simulink model "TraditionalStarterGenerator"  (R2024b)
settings: Solver=VariableStepAuto  StartTime=0.0  StopTime=20  MaxStep=1  RelTol=1e-3  EnableMultiTasking=on
undefined symbols (not defined in the file or in its folder): DiscIntNeverNeededParam
libraries: fl_lib x47, fl_ps_legacy_lib x26, ee_lib x25, nesl_utility x17, sdl_lib x1, SignalEditorBlockLib x1
(part 1 of 2)
CloseFcn:
  | try,close(h1_AutomotiveElectrical),end
  | clear h1_AutomotiveElectrical
  | 
  | clear simlog_AutomotiveElectrical
  | clear logsout_AutomotiveElectrical
  | clear tout
Description:
  | Automotive Electrical System
settings Model: Creator=The MathWorks, Inc.  LastModifiedBy=Ujjal.Ghosh
settings SolverCC: AlgebraicLoopSolver=TrustRegion  MaxZcPerStep=1
settings DataIOCC: LimitDataPoints=on  MaxDataPoints=15000  SaveFormat=Array  ReturnWorkspaceOutputs=off  SignalLoggingName=logsout_AutomotiveElectrical
settings OptimizationCC: ReuseModelBlockBuffer=off  ExpressionDepthLimit=2147483647  LifeSpan=inf
settings DebuggingCC: UnderspecifiedInitializationDetection=Classic  MergeDetectMultiDrivingBlocksExec=none  SolverPrmCheckMsg=warning  FcnCallInpInsideContextMsg=warning  UnconnectedInputMsg=warning  UnconnectedOutputMsg=warning  UnconnectedLineMsg=warning  AllowSymbolicDim=off  StateNameClashWarn=warning  SFUnexpectedBacktrackingDiag=warning  SFNoUnconditionalDefaultTransitionDiag=warning  SFExecutionAtInitializationDiag=none  ArithmeticOperatorsInVariantConditions=warning
settings HardwareCC: ProdBitPerPointer=32  ProdBitPerSizeT=32  ProdBitPerPtrDiffT=32  ProdLargestAtomicFloat=None  ProdIntDivRoundTo=Undefined  ProdEndianess=Unspecified  ProdWordSize=32  ProdHWDeviceType=32-bit Generic
settings ModelReferenceCC: EnableRefExpFcnMdlSchedulingChecks=on  PropagateSignalLabelsOutOfModel=off
settings SFSimCC: SimUseLocalCustomCode=off  CustomCodeUndefinedFunction=UseInterfaceOnly
settings RTWCC: RTWUseLocalCustomCode=off  GPUComputeCapability=3.5  DLArmComputeVersion=19.05
settings CodeAppCC: StateflowObjectComments=on
settings GRTTargetCC: TargetLangStandard=C89/C90 (ANSI)  CombineOutputUpdateFcns=off  GRTInterface=on
settings ConfigComp: CovMetricSettings=dw  CovSaveCumulativeToWorkspaceVar=on  CovSaveSingleToWorkspaceVar=on  CovExternalEMLEnable=off  CovSFcnEnable=off
settings SimscapeCC: SimscapeLogType=all  SimscapeLogSimulationStatistics=on  SimscapeLogName=simlog_AutomotiveElectrical  SimscapeLogDataHistory=15000

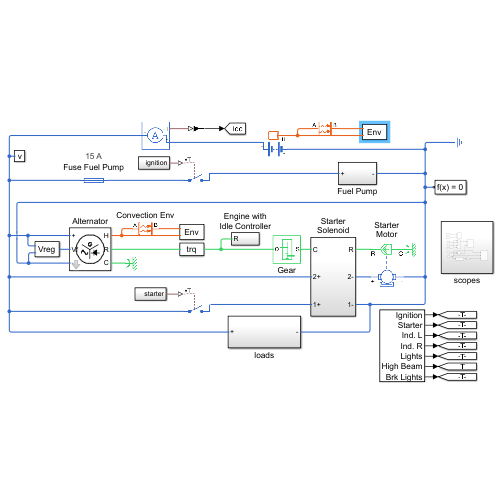
[thumbnail: Simulink's stored preview of the top-level diagram]
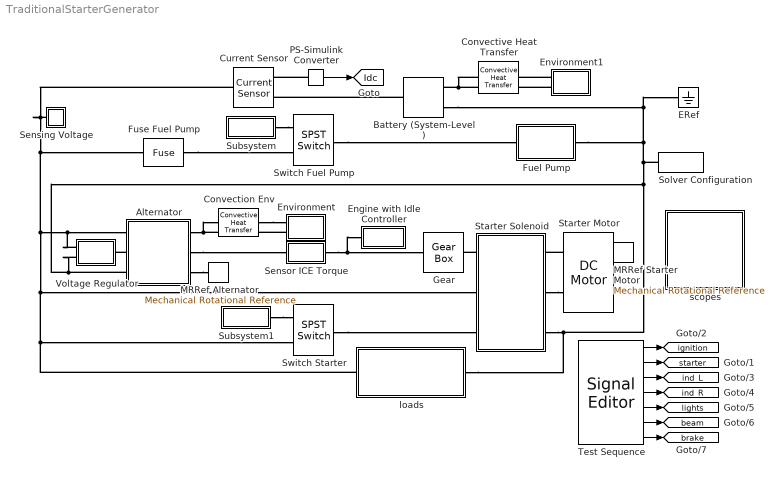
== system TraditionalStarterGenerator ==
  Alternator : Subsystem  mask(Abstracted Alternator){Kv=0.00125, Vmin=0.7, R=0.085, J=3*385, T0=25}
      mask prompts: Kv "Back emf constant (V/rpm)"; Vmin "Rectifier diode total forward voltage drop (V)"; R "Stator resistance represented on DC side (Ohm)"; J "Thermal mass (J/K)"; T0 "Initial temperature (deg C)"
      mask Display:
      | plot([287.470623152331;286.906458966957;285.219399620346;282.425692416244;278.552242282225;273.63635266052;267.725366255486;260.876209097478;253.154842314056;244.635626888274;235.40060752176;225.538722499386;215.144947164975;204.319379256811;193.166274911708;181.793044621416;170.309218810871;158.825393000326;147.452162710034;136.299058364931;125.473490456767;115.079715122356;105.217830099983;95.9828107334681;87.4635953076864;79.7422285242648;72.8930713662563;66.9820849612226;62.066195339518;58.1927452054981;55.3990380013969;53.7119786547854;53.147814469412;53.7119786547854;55.3990380013969;58.1927452054983;62.0661953395182;66.9820849612228;72.8930713662566;79.7422285242652;87.4635953076867;95.9828107334684;105.217830099983;115.079715122356;125.473490456768;136.299058364931;147.452162710034;158.825393000326;170.309218810871;181.793044621417;193.166274911708;204.319379256811;215.144947164975;225.538722499386;235.40060752176;244.635626888274;253.154842314056;260.876209097477;267.725366255486;273.63635266052;278.552242282224;282.425692416244;285.219399620346;286.906458966957;287.470623152331;287.470623152331;287.470623152331], [170.309218810871;158.825393000326;147.452162710034;136.299058364931;125.473490456768;115.079715122356;105.217830099983;95.9828107334682;87.4635953076864;79.7422285242649;72.8930713662564;66.9820849612227;62.0661953395181;58.1927452054982;55.3990380013969;53.7119786547854;53.147814469412;53.7119786547854;55.3990380013969;58.1927452054982;62.0661953395181;66.9820849612227;72.8930713662565;79.742228524265;87.4635953076865;95.9828107334683;105.217830099983;115.079715122356;125.473490456768;136.299058364931;147.452162710034;158.825393000326;170.309218810872;181.793044621417;193.166274911709;204.319379256812;215.144947164975;225.538722499387;235.40060752176;244.635626888275;253.154842314056;260.876209097478;267.725366255486;273.63635266052;278.552242282225;282.425692416244;285.219399620346;286.906458966957;287.470623152331;286.906458966957;285.219399620346;282.425692416244;278.552242282225;273.63635266052;267.725366255486;260.876209097478;253.154842314056;244.635626888275;235.40060752176;225.538722499387;215.144947164975;204.319379256812;193.166274911709;181.793044621417;170.309218810872;170.309218810871;170.309218810871])
      | patch([5.6843418860808e-14;340.618437621743;340.618437621743;0;5.6843418860808e-14;0.472425017505941;0.472425017505941;340.146012604237;340.146012604237;0.472425017505941;5.6843418860808e-14], [340.618437621743;340.618437621743;0;5.6843418860808e-14;340.618437621743;340.146012604237;0.472425017505941;0.472425017505941;340.146012604237;340.146012604237;340.618437621743], [1;1;1])
      | plot([170.309218810871;170.309218810871], [170.309218810871;96.6109160799534])
      | plot([234.118091175333;170.309218810871], [207.15837017633;170.309218810871])
      | plot([169.868288794532;106.059416430071], [169.553338782862;206.465480150655])
      | plot([249.67662175186;181.647419231013], [141.963717760518;141.963717760518])
      | patch([227.000220911577;227.000220911577;204.323820071295;227.000220911577], [122.121867025271;161.805568495765;141.963717760518;122.121867025271], [0;0;0])
      | plot([227.000220911577;227.000220911577;204.323820071295;227.000220911577], [122.121867025271;161.805568495765;141.963717760518;122.121867025271])
      | plot([173.143768915907;184.481969336048], [204.323820071295;204.323820071295])
      | plot([204.323820071295;204.323820071295], [161.805568495765;122.121867025271])
      | plot([178.812869125977;178.749879123643;178.560909116641;178.308949107304;177.993999095634;177.490079076961;176.923169055954;176.356259034947;175.600379006937;174.844498978928;173.96263894625;172.89180890657;171.694998862222;170.309218810871;168.923438759521;167.600648710504;166.529818670824;165.710948640481;165.08104861714;164.577128598467;164.136198582128;163.758258568123;163.317328551784;162.687428528443;161.994538502768;161.049688467756;160.04184843041;158.97101839073;157.90018835105;157.207298325375;156.703378306702;156.451418297365;156.388428295031;156.388428295031;156.388428295031;156.388428295031;156.388428295031;156.325438292697;156.199458288029;156.136468285695;156.199458288029;156.325438292697;156.388428295031;156.388428295031;156.388428295031;156.388428295031;156.388428295031;156.451418297365;156.703378306702;157.207298325375;157.90018835105;158.97101839073;160.04184843041;161.049688467756;161.994538502768;162.687428528443;163.317328551784;163.758258568123;164.199188584462;164.577128598467;165.08104861714;165.710948640481;166.529818670824;167.600648710504;168.923438759521;170.309218810871;171.883968869224;173.143768915907;174.088618950918;174.781508976594;175.159448990598;175.537389004603;175.78934901394;176.167289027944;176.608219044283;177.238119067624;178.056989097968;178.812869125977;179.190809139982;179.442769149318;179.631739156321;179.757719160989;179.883699165657;179.883699165657;179.883699165657;179.883699165657;179.820709163323;179.694729158655;179.631739156321;179.505759151653;179.379779146984;179.253799142316;179.127819137648;179.064829135314;178.938849130645;178.875859128311;178.812869125977], [218.496570596471;218.62255060114;218.811520608142;219.189460622147;219.69338064082;220.323280664161;220.953180687502;221.646070713177;222.275970736519;222.842880757526;223.346800776199;223.787730792537;224.039690801874;224.165670806542;224.039690801874;223.850720794872;223.535770783201;223.283810773864;223.031850764528;222.779890755192;222.527930745855;222.212980734184;221.898030722514;221.520090708509;220.953180687502;220.323280664161;219.441420631483;218.496570596471;217.299760552123;216.291920514777;215.536040486768;215.032120468095;214.717170456424;214.465210447088;214.213250437751;213.898300426081;213.331390405074;212.51252037473;211.378700332716;209.992920281366;208.607140230015;207.473320188001;206.654450157657;206.08754013665;205.77259012498;205.520630115643;205.268670106307;204.953720094636;204.449800075963;203.693920047954;202.686080010608;201.48926996626;200.544419931248;199.66255989857;199.032659875229;198.465749854222;198.087809840217;197.772859828547;197.457909816876;197.20594980754;196.953989798203;196.702029788867;196.45006977953;196.13511976786;195.946149760857;195.820169756189;195.946149760857;196.261099772528;196.702029788867;197.079969802871;197.52089981921;197.961829835549;198.402759851888;198.906679870561;199.410599889234;200.040499912575;200.73338993825;201.48926996626;201.867209980264;202.182159991935;202.497110003606;202.749070012942;203.001030022278;203.190000029281;203.378970036283;203.504950040951;203.63093004562;203.756910050288;203.882890054956;203.94588005729;204.071860061958;204.134850064293;204.197840066627;204.260830068961;204.260830068961;204.323820071295;204.323820071295])
      | plot([98.8785561639816;98.9415461663157;99.0045361686498;99.1935061756522;99.5084561873228;99.8863962013275;100.327326217666;100.831246236339;101.46114625968;102.091046283022;102.783936308697;103.60280633904;104.421676369384;105.366526404396;106.374366441742;107.57117648609;108.830976532772;110.216756584123;111.602536635473;112.92532668449;114.059146726504;115.003996761516;115.696886787191;116.200806805864;116.578746819869;116.830706829205;117.082666838542;117.271636845544;117.586586857215;117.964526871219;118.531436892226;119.224326917902;120.232166955248;121.428976999596;122.814757050946;124.389507109299;125.964257167652;127.350037219003;128.546847263351;129.554687300697;130.247577326372;130.814487347379;131.192427361384;131.507377373055;131.696347380057;131.948307389394;132.20026739873;132.578207412735;133.082127431408;133.775017457083;134.719867492095;135.853687534109;137.176477583125;138.562257634476;139.948037685826;141.207837732509;142.404647776857;143.412487814203;144.357337849215;145.176207879558;145.995077909902;146.687967935577;147.317867958918;147.947767982259;148.451688000932;148.892618017271;149.270558031276;149.585508042947;149.774478049949;149.837468052283;149.900458054617], [141.522787744179;141.711757751182;142.089697765186;142.782587790862;143.790427828208;145.05022787489;146.561987930909;148.199727991596;149.963448056951;151.727168122307;153.427898185328;155.065638246015;156.640388304368;158.026168355718;159.222978400067;160.230818437412;160.986698465422;161.364638479427;161.301648477092;160.923708463088;160.356798442081;159.663908416405;158.97101839073;158.215138362721;157.459258334711;156.703378306702;155.947498278692;155.128628248349;154.246768215671;153.301918180659;152.231088140979;151.034278096631;149.585508042947;148.010757984594;146.247037919238;144.357337849215;142.467637779191;140.703917713836;139.129167655483;137.743387604132;136.546577559784;135.475747520104;134.593887487426;133.775017457083;133.019137429074;132.326247403398;131.570367375389;130.877477349714;130.121597321704;129.365717293695;128.672827268019;127.979937242344;127.539007226005;127.350037219003;127.539007226005;128.105917247012;128.924787277356;129.932627314702;131.12943735905;132.452227408066;133.838007459417;135.349767515436;136.924517573789;138.436277629808;139.948037685826;141.270827734843;142.341657774523;143.223517807201;143.853417830542;144.168367842212;144.357337849215])
  Battery (System-Level) : sdl_lib/Sources/Battery (System-Level)  Vnom=12 V  R1=35 mOhm  prm_AH=sdl.enum.InfiniteFinite.Finite  AH=3 A*hr  V1=11.8 V  AH1=0.3 A*hr  prm_R2=sdl.enum.DisabledEnabled.Disabled  R2=2000 Ohm  thermal_port=simscape.enum.thermaleffects.model  thermal_mass=420 J/K  i_specify=off  i_priority=None  i=0 A  i_nominal_specify=off  i_nominal_value=1  i_nominal_unit=A  v_specify=off  v_priority=None  v=0 V  v_nominal_specify=off  v_nominal_value=1  v_nominal_unit=V  charge_specify=on  charge_priority=High  charge=1.5 A*hr  charge_nominal_specify=off  charge_nominal_value=1  charge_nominal_unit=A*hr  temperature_specify=on  temperature_priority=Low  temperature=25 degC  temperature_nominal_specify=off  temperature_nominal_value=1  temperature_nominal_unit=K
      settings: InternalSimscapePortConfiguration="{\"Bottom\":[],\"Left\":[{\"id\":\"p\",\"label\":\"+\",\"type\":\"foundation.electrical.electrical\"}],\"Right\":[{\"id\":\"n\",\"label\":\"-\",\"type\":\"foundation.electrical.electrical\"},{\"id\":\"H\",\"label\":\"H\",\"type\":\"foundation.thermal.thermal\"}],\"Top\":[]}"
  Convection Env : fl_lib/Thermal/Thermal Elements/Convective Heat Transfer  thermal_type=foundation.enum.constant_variable.constant  area=0.01 m^2  heat_tr_coeff=100 W/(m^2 * K)  min_heat_tr_coeff=1e-3 W/(K*m^2)  T_specify=off  T_priority=High  T=0 K  T_nominal_specify=off  T_nominal_value=1  T_nominal_unit=K  Q_specify=off  Q_priority=High  Q=0 J/s  Q_nominal_specify=off  Q_nominal_value=1  Q_nominal_unit=J/s
  Convective Heat Transfer : fl_lib/Thermal/Thermal Elements/Convective Heat Transfer  thermal_type=foundation.enum.constant_variable.constant  area=0.02 m^2  heat_tr_coeff=20 W/(m^2*K)  min_heat_tr_coeff=20 W/(K*m^2)  T_specify=off  T_priority=None  T=0 K  T_nominal_specify=off  T_nominal_value=1  T_nominal_unit=K  Q_specify=off  Q_priority=None  Q=0 W  Q_nominal_specify=off  Q_nominal_value=1  Q_nominal_unit=W
  Current Sensor : fl_lib/Electrical/Electrical Sensors/Current Sensor
  ERef : fl_lib/Electrical/Electrical Elements/Electrical Reference
  Engine with Idle Controller : Subsystem
  Environment : Subsystem
      mask Display: disp('Env')
  Environment1 : Subsystem
      mask Display: disp('Env')
  Fuel Pump : Subsystem
  Fuse Fuel Pump : ee_lib/Switches & Breakers/Fuse  prm=1  I_rated=15 A  melt_margin=1  T_fuse=0.5 s  I2t=1 s*A^2  I_vec=[1.9, 2.0, 2.5, 30.0] A  t_vec=[10000.0, 1.0, 0.3, 0.001] s  R_closed=0.01 Ohm  G_open=1e-8 1/Ohm  exposemeasurement=ee.enum.exposemeasurement.hidden
      settings: AttributesFormatString=%<I_rated> %<I_rated_unit>  InternalSimscapePortConfiguration="{\"Bottom\":[],\"Left\":[{\"id\":\"p\",\"label\":\"\",\"type\":\"foundation.electrical.electrical\"}],\"Right\":[{\"id\":\"n\",\"label\":\"\",\"type\":\"foundation.electrical.electrical\"}],\"Top\":[]}"
  Gear : fl_lib/Mechanical/Mechanisms/Gear Box  ratio=5  t_in_specify=off  t_in_priority=High  t_in=0 N*m  t_in_nominal_specify=off  t_in_nominal_value=1  t_in_nominal_unit=N*m  t_out_specify=off  t_out_priority=High  t_out=0 N*m  t_out_nominal_specify=off  t_out_nominal_value=1  t_out_nominal_unit=N*m
  MRRef Alternator : fl_lib/Mechanical/Rotational Elements/Mechanical Rotational Reference
  MRRef Starter Motor : fl_lib/Mechanical/Rotational Elements/Mechanical Rotational Reference
  PS-Simulink Converter : nesl_utility/PS-Simulink Converter  PhysicalDomain=network_engine_domain  SubClassName=ps_output  LeftPortType=input  RightPortType=output  PseudoPeriodic=off  Frequencies=[]  VectorFormat=inherit  Unit=inherit  AffineConversion=off
  Sensing Voltage : Subsystem
      mask Display: disp('v')
  Sensor ICE Torque : Subsystem
      mask Display: disp('trq')
  Solver Configuration : nesl_utility/Solver Configuration  PhysicalDomain=network_engine_domain  SubClassName=solver  LeftPortType=input  RightPortType=generic  Tones=[]  Harmonics=[]  SimulateNoise=on  Profile=off  UseLocalSampling=off  EnableSwitchedLinearOptims=on  FrequencyDomain=off  UseCCode=off  RelTol=0.001  AbsTol=1e-06  MinStep=1e-09  ToWorkspace=off  RevertToSquareIcSolve=off  NumHomotopyIterations=100  PhasorMode=off  PhasorModeNumHarmonics=1  ConsistencySolver=NEWTON_FTOL  IndexReductionMethod=DerivativeReplacement  DoDC=off  ResidualTolerance=1e-9  ConsistencyTolSource=GLOBAL  ConsistencyAbsTol=0.001  ConsistencyRelTol=0.001  ConsistencyTolFactor=0.001  UseLocalSolver=on  LocalSolverChoice=NE_TRAPEZOIDAL_ADVANCER  ResolveIndetEquations=on  FunctionEvalNumThread=1  LocalSolverSampleTime=0.002  DoFixedCost=on  MaxNonlinIter=10  MaxModeIter=2  ComputeImpulses=off  ImpulseIterations=2  LinearAlgebra=auto  LinearAlgebraNumThread=0  EquationFormulation=NE_TIME_EF  DelaysMemoryBudget=1024  AutomaticFiltering=on  FilteringTimeConstant=0.001  PartitionStorageMethod=AS_NEEDED  PartitionMemoryBudget=1024  PartitionMethod=FAST  MultibodyUseLocalSolver=off  MultibodyLocalSolverChoice=ODE1  MultibodyLocalSolverSampleTime=0.001
  Starter Motor : ee_lib/Electromechanical/Brushed Motors/DC Motor  field_option=ee.enum.field_option.pm  Rf=100 Ohm  Lf=1 H  Laf=0.15 H  If0=0 A  parameterization=2  Ra=3.9 Ohm  La=1 mH  emf_or_torque=1  Kv=7.2e-5 V/rpm  Ki=6.876e-4 N*m/A  T_stall=3.5 N*m  w_max=6000 rpm  w_rated=1.5e+4 rpm  P_rated=0.08 W  V_rated=12 V  lam_param=1  i_noload=0 A  V_i_noload=1.5 V  J=0.001 kg*m^2  lam=0 N*m/(rad/s)  speed0=0 rpm  t_fault_armature=1 s  t_fault_field=1 s  fault_action=simscape.enum.assert.action.none  alpha=3.93e-3 1/K  Tmeas=25 degC  thermal_mass=100 J/K  initial_temperature=25 degC
  Starter Solenoid : Subsystem  Tag=PublishSubsystem
  Subsystem : Subsystem
  Subsystem1 : Subsystem
  Switch Fuel Pump : ee_lib/Switches & Breakers/SPST Switch  R_closed=1 Ohm  G_open=1e-6 S  Threshold=0.5 V  Width=0 V  model_dynamics=0  t_on=0.001 s  t_off=0.001 s  initial_vT=0 V
      settings: InternalSimscapePortConfiguration="{\"Bottom\":[],\"Left\":[{\"id\":\"vT\",\"label\":\"vT\",\"type\":\"input\"},{\"id\":\"p\",\"label\":\"\",\"type\":\"foundation.electrical.electrical\"}],\"Right\":[{\"id\":\"n\",\"label\":\"\",\"type\":\"foundation.electrical.electrical\"}],\"Top\":[]}"
  Switch Starter : ee_lib/Switches & Breakers/SPST Switch  R_closed=1 Ohm  G_open=1e-6 S  Threshold=0.5 V  Width=0 V  model_dynamics=0  t_on=0.001 s  t_off=0.001 s  initial_vT=0 V
      settings: InternalSimscapePortConfiguration="{\"Bottom\":[],\"Left\":[{\"id\":\"vT\",\"label\":\"vT\",\"type\":\"input\"},{\"id\":\"p\",\"label\":\"\",\"type\":\"foundation.electrical.electrical\"}],\"Right\":[{\"id\":\"n\",\"label\":\"\",\"type\":\"foundation.electrical.electrical\"}],\"Top\":[]}"
  Test Sequence : SignalEditorBlockLib/Signal Editor  FileName=C:\Users\Ujjal.Ghosh\Documents\MATLAB\Examples\R2024b\simscapeelectrical\AutomotiveElectricalExample\AutomotiveElectricalTestSequence.mat  ActiveScenario=Start_lights_off  ActiveSignal=Brk Lights  IsBus=off  OutputBusObjectStr=Bus: BusObject  SampleTime=0  OutputAfterFinalValue=Extrapolation  Unit=inherit  PreserveSignalName=on  ApplySigPropsToAllScenarios=on  ApplySigPropsToAllSignals=off
  Voltage Regulator : Subsystem
      mask Display: disp('Vreg')
  loads : Subsystem  Tag=PublishSubsystem
  scopes : Subsystem
  tag scope: Idc=global, beam=global, brake=global, ignition=global, ind_L=global, ind_R=global, lights=global, starter=global
  wires:
  Test Sequence/1 -> [ignition]
  Test Sequence/2 -> [starter]
  Test Sequence/3 -> [ind_L]
  Test Sequence/4 -> [ind_R]
  Test Sequence/5 -> [lights]
  Test Sequence/6 -> [beam]
  Test Sequence/7 -> [brake]
  PS-Simulink Converter/1 -> [Idc]
  connections:
  Convection Env/RConn1 -- Environment/LConn1
  MRRef Starter Motor/LConn1 -- Starter Motor/RConn2
  Starter Solenoid/RConn2 -- Starter Motor/LConn1
  Engine with Idle Controller/LConn1 -- Sensor ICE Torque/LConn1 -- Gear/RConn1
  Starter Motor/LConn2 -- Starter Solenoid/RConn1
  Starter Solenoid/LConn1 -- Gear/LConn1
  Fuse Fuel Pump/RConn1 -- Switch Fuel Pump/LConn2
  Switch Fuel Pump/RConn1 -- Fuel Pump/LConn1
  Subsystem/RConn1 -- Switch Fuel Pump/LConn1
  Switch Starter/RConn1 -- Starter Solenoid/LConn3
  Subsystem1/RConn1 -- Switch Starter/LConn1
  Current Sensor/LConn1 -- Sensing Voltage/LConn1 -- Fuse Fuel Pump/LConn1 -- loads/RConn1 -- Switch Starter/LConn2 -- Starter Solenoid/LConn2 -- Alternator/LConn1 -- Voltage Regulator/LConn1
  ERef/LConn1 -- Battery (System-Level)/RConn1 -- Fuel Pump/RConn1 -- Solver Configuration/RConn1 -- Alternator/LConn3 -- Voltage Regulator/LConn2 -- Starter Motor/RConn1 -- loads/LConn1 -- Starter Solenoid/RConn3
  Alternator/RConn3 -- MRRef Alternator/LConn1
  Alternator/LConn2 -- Voltage Regulator/RConn1
  Alternator/RConn1 -- Convection Env/LConn1 -- Environment/LConn2
  Alternator/RConn2 -- Sensor ICE Torque/RConn1
  Battery (System-Level)/LConn1 -- Current Sensor/RConn2
  PS-Simulink Converter/LConn1 -- Current Sensor/RConn1
  Convective Heat Transfer/LConn1 -- Environment1/LConn2 -- Battery (System-Level)/RConn2
  Environment1/LConn1 -- Convective Heat Transfer/RConn1

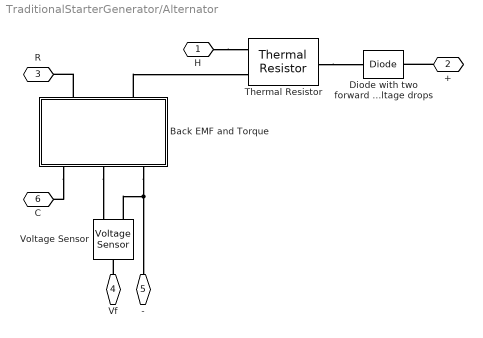
== system TraditionalStarterGenerator/Alternator ==
  Back EMF and Torque : Subsystem
  Diode with two forward voltage drops : fl_lib/Electrical/Electrical Elements/Diode  Vf=Vmin V  Ron=0.01*R Ohm  Goff=1e-5 1/Ohm  i_specify=off  i_priority=High  i=0 A  i_nominal_specify=off  i_nominal_value=1  i_nominal_unit=A  v_specify=off  v_priority=High  v=0 V  v_nominal_specify=off  v_nominal_value=1  v_nominal_unit=V
  Thermal Resistor : fl_lib/Electrical/Electrical Elements/Thermal Resistor  R0=0.99*R Ohm  T0=25 degC  alpha=5e-5 1/K  tc=100 s  K_d=J/100 W/K  T_specify=on  T_priority=High  T=T0 degC  T_nominal_specify=off  T_nominal_value=1  T_nominal_unit=K
      settings: InternalSimscapePortConfiguration="{\"Bottom\":[],\"Left\":[{\"id\":\"H\",\"label\":\"H\",\"type\":\"foundation.thermal.thermal\"},{\"id\":\"p\",\"label\":\"+\",\"type\":\"foundation.electrical.electrical\"}],\"Right\":[{\"id\":\"n\",\"label\":\"-\",\"type\":\"foundation.electrical.electrical\"}],\"Top\":[]}"
  Voltage Sensor : fl_lib/Electrical/Electrical Sensors/Voltage Sensor
  H : PMIOPort  Side=Right
  + : PMIOPort  Port=2  Side=Left
  R : PMIOPort  Port=3  Side=Right
  Vf : PMIOPort  Port=4  Side=Left
  - : PMIOPort  Port=5  Side=Left
  C : PMIOPort  Port=6  Side=Right
  connections:
  Back EMF and Torque/RConn3 -- Voltage Sensor/RConn2 -- -/RConn1
  Back EMF and Torque/LConn2 -- Thermal Resistor/LConn2
  Thermal Resistor/RConn1 -- Diode with two forward voltage drops/LConn1
  Vf/RConn1 -- Voltage Sensor/LConn1
  +/RConn1 -- Diode with two forward voltage drops/RConn1
  H/RConn1 -- Thermal Resistor/LConn1
  Back EMF and Torque/LConn1 -- R/RConn1
  Back EMF and Torque/RConn2 -- Voltage Sensor/RConn1
  Back EMF and Torque/RConn1 -- C/RConn1

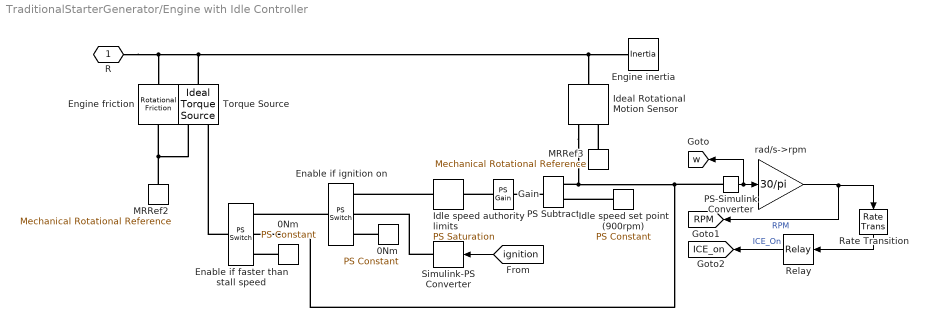
== system TraditionalStarterGenerator/Engine with Idle Controller ==
  " 0Nm " : fl_lib/Physical Signals/Sources/PS Constant  constant=0
  0Nm : fl_lib/Physical Signals/Sources/PS Constant  constant=0
  Enable if faster than stall speed : fl_ps_legacy_lib/Legacy Physical Signals/Nonlinear Operators/PS Switch  Threshold=700*2*pi/60
      settings: InternalSimscapePortConfiguration="{\"Bottom\":[],\"Left\":[{\"id\":\"I1\",\"label\":\"\",\"type\":\"input\"},{\"id\":\"I2\",\"label\":\"\",\"type\":\"input\"},{\"id\":\"I3\",\"label\":\"\",\"type\":\"input\"}],\"Right\":[{\"id\":\"O\",\"label\":\"\",\"type\":\"output\"}],\"Top\":[]}"
  Enable if ignition on : fl_ps_legacy_lib/Legacy Physical Signals/Nonlinear Operators/PS Switch  Threshold=0.5
      settings: InternalSimscapePortConfiguration="{\"Bottom\":[],\"Left\":[{\"id\":\"I1\",\"label\":\"\",\"type\":\"input\"},{\"id\":\"I2\",\"label\":\"\",\"type\":\"input\"},{\"id\":\"I3\",\"label\":\"\",\"type\":\"input\"}],\"Right\":[{\"id\":\"O\",\"label\":\"\",\"type\":\"output\"}],\"Top\":[]}"
  Engine friction : fl_lib/Mechanical/Rotational Elements/Rotational Friction  brkwy_trq=2.5 N*m  brkwy_vel=0.060623 rad/s  Col_trq=2 N*m  visc_coef=0.00001 N*m/(rad/s)  w_specify=off  w_priority=High  w=0 rad/s  w_nominal_specify=off  w_nominal_value=1  w_nominal_unit=rad/s  t_specify=off  t_priority=High  t=0 N*m  t_nominal_specify=off  t_nominal_value=1  t_nominal_unit=N*m
  Engine inertia : fl_lib/Mechanical/Rotational Elements/Inertia  inertia=0.05 kg*m^2  num_ports=foundation.enum.numPorts2.one  w_specify=on  w_priority=High  w=0 rad/s  w_nominal_specify=off  w_nominal_value=1  w_nominal_unit=rad/s  t_specify=off  t_priority=High  t=0 N*m  t_nominal_specify=off  t_nominal_value=1  t_nominal_unit=N*m
  Gain : fl_ps_legacy_lib/Legacy Physical Signals/Functions/PS Gain  gain=5
  Ideal Rotational Motion Sensor : fl_lib/Mechanical/Mechanical Sensors/Ideal Rotational Motion Sensor  reference=foundation.enum.MeasurementReference.difference  acceleration_port=false  velocity_port=true  position_port=false  wrap_angle=simscape.enum.onoff.off  offset=0 rad
      settings: InternalSimscapePortConfiguration="{\"Bottom\":[],\"Left\":[{\"id\":\"R\",\"label\":\"R\",\"type\":\"foundation.mechanical.rotational.rotational\"}],\"Right\":[{\"id\":\"C\",\"label\":\"C\",\"type\":\"foundation.mechanical.rotational.rotational\"},{\"id\":\"W\",\"label\":\"W\",\"type\":\"output\"}],\"Top\":[]}"
  Idle speed authority limits : fl_ps_legacy_lib/Legacy Physical Signals/Nonlinear Operators/PS Saturation  upper_limit=6.5  lower_limit=0
      settings: InternalSimscapePortConfiguration="{\"Bottom\":[],\"Left\":[{\"id\":\"I\",\"label\":\"\",\"type\":\"input\"}],\"Right\":[{\"id\":\"O\",\"label\":\"\",\"type\":\"output\"}],\"Top\":[]}"
  Idle speed set point (900rpm) : fl_lib/Physical Signals/Sources/PS Constant  constant=900*2*pi/60
  MRRef2 : fl_lib/Mechanical/Rotational Elements/Mechanical Rotational Reference
  MRRef3 : fl_lib/Mechanical/Rotational Elements/Mechanical Rotational Reference
  PS Subtract : fl_ps_legacy_lib/Legacy Physical Signals/Functions/PS Subtract
  PS-Simulink Converter : nesl_utility/PS-Simulink Converter  PhysicalDomain=network_engine_domain  SubClassName=ps_output  LeftPortType=input  RightPortType=output  PseudoPeriodic=off  Frequencies=[]  VectorFormat=1-D array  Unit=rad/s  AffineConversion=off
  Rate Transition : RateTransition  OutPortSampleTime=0.0001
  Relay : Relay  OnSwitchValue=850  OffSwitchValue=500  ZeroCross=off
  Simulink-PS Converter : nesl_utility/Simulink-PS Converter  PhysicalDomain=network_engine_domain  SubClassName=ps_input  LeftPortType=input  RightPortType=output  PseudoPeriodic=off  Frequencies=[]  NoiseDistribution=none  NoiseParameters=[]  Unit=1  AffineConversion=off  FilteringAndDerivatives=zero  SimscapeFilterOrder=1  InputFilterTimeConstant=0.001  UdotUserProvided=1
  Torque Source : fl_lib/Mechanical/Mechanical Sources/Ideal Torque Source
  rad/s->rpm : Gain  Gain=30/pi
  R : PMIOPort  Side=Left
  tag scope: ICE_on=global, RPM=global, w=global
  wires:
  [ignition] -> Simulink-PS Converter/1
  rad/s->rpm/1 -> [RPM], Rate Transition/1  "RPM"
  PS-Simulink Converter/1 -> [w], rad/s->rpm/1
  Rate Transition/1 -> Relay/1
  Relay/1 -> [ICE_on]  "ICE_On"
  connections:
  R/RConn1 -- Engine inertia/LConn1 -- Ideal Rotational Motion Sensor/LConn1 -- Torque Source/LConn1 -- Engine friction/LConn1
  MRRef2/LConn1 -- Torque Source/RConn2 -- Engine friction/RConn1
  Ideal Rotational Motion Sensor/RConn2 -- Enable if faster than stall speed/LConn2 -- PS-Simulink Converter/LConn1 -- PS Subtract/LConn2
  Idle speed set point (900rpm)/RConn1 -- PS Subtract/LConn1
  Idle speed authority limits/RConn1 -- Enable if ignition on/LConn1
  0Nm/RConn1 -- Enable if ignition on/LConn3
  MRRef3/LConn1 -- Ideal Rotational Motion Sensor/RConn1
  PS Subtract/RConn1 -- Gain/LConn1
  Gain/RConn1 -- Idle speed authority limits/LConn1
  Simulink-PS Converter/RConn1 -- Enable if ignition on/LConn2
  Enable if ignition on/RConn1 -- Enable if faster than stall speed/LConn1
  Enable if faster than stall speed/RConn1 -- Torque Source/RConn1
  " 0Nm "/RConn1 -- Enable if faster than stall speed/LConn3

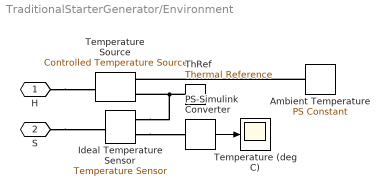
== system TraditionalStarterGenerator/Environment ==
  " Temperature Source" : fl_lib/Thermal/Thermal Sources/Controlled Temperature Source
  Ambient Temperature : fl_lib/Physical Signals/Sources/PS Constant  constant=298.15
  Ideal Temperature Sensor : fl_lib/Thermal/Thermal Sensors/Temperature Sensor  temperature_measure=foundation.enum.MeasurementReference.difference
  PS-Simulink Converter : nesl_utility/PS-Simulink Converter  PhysicalDomain=network_engine_domain  SubClassName=ps_output  LeftPortType=input  RightPortType=output  PseudoPeriodic=off  Frequencies=[]  VectorFormat=1-D array  Unit=degC  AffineConversion=on
  Temperature (deg C) : Scope
  ThRef : fl_lib/Thermal/Thermal Elements/Thermal Reference
  H : PMIOPort  Side=Left
  S : PMIOPort  Port=2  Side=Left
  wires:
  PS-Simulink Converter/1 -> Temperature (deg C)/1
  connections:
  Ambient Temperature/RConn1 -- " Temperature Source"/RConn1
  H/RConn1 -- " Temperature Source"/LConn1
  ThRef/LConn1 -- Ideal Temperature Sensor/RConn1 -- " Temperature Source"/RConn2
  Ideal Temperature Sensor/RConn2 -- PS-Simulink Converter/LConn1
  S/RConn1 -- Ideal Temperature Sensor/LConn1

== system TraditionalStarterGenerator/Environment1 ==
  " Temperature Source" : fl_lib/Thermal/Thermal Sources/Controlled Temperature Source
  Ambient Temperature : fl_lib/Physical Signals/Sources/PS Constant  constant=298.15
  Ideal Temperature Sensor : fl_lib/Thermal/Thermal Sensors/Temperature Sensor  temperature_measure=foundation.enum.MeasurementReference.difference
  PS-Simulink Converter : nesl_utility/PS-Simulink Converter  PhysicalDomain=network_engine_domain  SubClassName=ps_output  LeftPortType=input  RightPortType=output  PseudoPeriodic=off  Frequencies=[]  VectorFormat=1-D array  Unit=degC  AffineConversion=on
  Temperature (deg C) : Scope
  ThRef : fl_lib/Thermal/Thermal Elements/Thermal Reference
  H : PMIOPort  Side=Left
  S : PMIOPort  Port=2  Side=Left
  wires:
  PS-Simulink Converter/1 -> Temperature (deg C)/1
  connections:
  Ambient Temperature/RConn1 -- " Temperature Source"/RConn1
  H/RConn1 -- " Temperature Source"/LConn1
  ThRef/LConn1 -- Ideal Temperature Sensor/RConn1 -- " Temperature Source"/RConn2
  Ideal Temperature Sensor/RConn2 -- PS-Simulink Converter/LConn1
  S/RConn1 -- Ideal Temperature Sensor/LConn1

== system TraditionalStarterGenerator/Fuel Pump ==
  Resistive Load : fl_lib/Electrical/Electrical Elements/Resistor  R=5 Ohm  i_specify=off  i_priority=High  i=0 A  i_nominal_specify=off  i_nominal_value=1  i_nominal_unit=A  v_specify=off  v_priority=High  v=0 V  v_nominal_specify=off  v_nominal_value=1  v_nominal_unit=V
  + : PMIOPort  Side=Left
  - : PMIOPort  Port=2  Side=Right
  connections:
  Resistive Load/RConn1 -- -/RConn1
  +/RConn1 -- Resistive Load/LConn1

== system TraditionalStarterGenerator/Sensing Voltage ==
  Battery Voltage : nesl_utility/PS-Simulink Converter  PhysicalDomain=network_engine_domain  SubClassName=ps_output  LeftPortType=input  RightPortType=output  PseudoPeriodic=off  Frequencies=[]  VectorFormat=1-D array  Unit=1  AffineConversion=off
  ERef : fl_lib/Electrical/Electrical Elements/Electrical Reference
  Voltage Sensor : fl_lib/Electrical/Electrical Sensors/Voltage Sensor
  + : PMIOPort  Side=Left
  tag scope: Vdc=global
  wires:
  Battery Voltage/1 -> [Vdc]  "Battery Voltage"
  connections:
  Voltage Sensor/LConn1 -- +/RConn1
  Battery Voltage/LConn1 -- Voltage Sensor/RConn1
  ERef/LConn1 -- Voltage Sensor/RConn2

== system TraditionalStarterGenerator/Sensor ICE Torque ==
  PS-Simulink Converter3 : nesl_utility/PS-Simulink Converter  PhysicalDomain=network_engine_domain  SubClassName=ps_output  LeftPortType=input  RightPortType=output  PseudoPeriodic=off  Frequencies=[]  VectorFormat=1-D array  Unit=N*m  AffineConversion=off
  Torque Sensor : fl_lib/Mechanical/Mechanical Sensors/Ideal Torque Sensor
  R : PMIOPort  Side=Left
  C : PMIOPort  Port=2  Side=Right
  tag scope: tq=global
  wires:
  PS-Simulink Converter3/1 -> [tq]
  connections:
  Torque Sensor/RConn2 -- PS-Simulink Converter3/LConn1
  C/RConn1 -- Torque Sensor/RConn1
  R/RConn1 -- Torque Sensor/LConn1

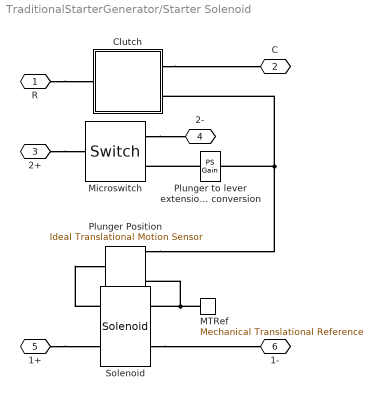
== system TraditionalStarterGenerator/Starter Solenoid ==
  Clutch : Subsystem
  MTRef : fl_lib/Mechanical/Translational Elements/Mechanical Translational Reference
  Microswitch : fl_lib/Electrical/Electrical Elements/Switch  R_closed=0.01 Ohm  G_open=1e-8 1/Ohm  Threshold=-2e-3  i_specify=off  i_priority=High  i=0 A  i_nominal_specify=off  i_nominal_value=1  i_nominal_unit=A  v_specify=off  v_priority=High  v=0 V  v_nominal_specify=off  v_nominal_value=1  v_nominal_unit=V
  Plunger Position : fl_lib/Mechanical/Mechanical Sensors/Ideal Translational Motion Sensor  reference=foundation.enum.MeasurementReference.difference  acceleration_port=false  velocity_port=true  position_port=true  offset=10 mm
  Plunger to lever extension conversion : fl_ps_legacy_lib/Legacy Physical Signals/Functions/PS Gain  gain=-1
  Solenoid : ee_lib/Electromechanical/Mechatronic Actuators/Solenoid  motionDirection=ee.enum.actuators.solenoidDirection.towards  F12=[ 45 5 ] N  X12=[ 2 10 ] mm  Vdc=12 V  Imax=2 A  K=200 N/m  Xzero=10 mm  lam=5 N/(m/s)  Mass=0.5 kg  Xmax=Inf mm  K_endstop=1e+6 N/m  D_endstop=500 N/(m/s)  i_specify=off  i_priority=High  i=0 A  i_nominal_specify=off  i_nominal_value=1  i_nominal_unit=A  x_specify=on  x_priority=High  x=10 mm  x_nominal_specify=off  x_nominal_value=1  x_nominal_unit=mm  vel_specify=off  vel_priority=None  vel=0 m/s  vel_nominal_specify=off  vel_nominal_value=1  vel_nominal_unit=m/s  F_specify=off  F_priority=None  F=0 N  F_nominal_specify=off  F_nominal_value=1  F_nominal_unit=N  v_L_specify=off  v_L_priority=None  v_L=0 V  v_L_nominal_specify=off  v_L_nominal_value=1  v_L_nominal_unit=V  magnetic_force_specify=off  magnetic_force_priority=None  magnetic_force=0 N  magnetic_force_nominal_specify=off  magnetic_force_nominal_value=1  magnetic_force_nominal_unit=N  alpha=3.93e-3 1/K  Tmeas=25 degC  thermal_mass=100 J/K  temperature_specify=off  temperature_priority=High  temperature=25 degC  temperature_nominal_specify=off  temperature_nominal_value=1  temperature_nominal_unit=degC  Q_specify=off  Q_priority=None  Q=0 W  Q_nominal_specify=off  Q_nominal_value=1  Q_nominal_unit=W
      settings: InternalSimscapePortConfiguration="{\"Bottom\":[],\"Left\":[{\"id\":\"p\",\"label\":\"+\",\"type\":\"foundation.electrical.electrical\"},{\"id\":\"R\",\"label\":\"R\",\"type\":\"foundation.mechanical.translational.translational\"}],\"Right\":[{\"id\":\"n\",\"label\":\"-\",\"type\":\"foundation.electrical.electrical\"},{\"id\":\"C\",\"label\":\"C\",\"type\":\"foundation.mechanical.translational.translational\"}],\"Top\":[]}"
  R : PMIOPort  Side=Right
  C : PMIOPort  Port=2  Side=Left
  2+ : PMIOPort  Port=3  Side=Left
  2- : PMIOPort  Port=4  Side=Right
  1+ : PMIOPort  Port=5  Side=Left
  1- : PMIOPort  Port=6  Side=Right
  connections:
  1+/RConn1 -- Solenoid/LConn1
  Solenoid/RConn1 -- 1-/RConn1
  MTRef/LConn1 -- Solenoid/RConn2 -- Plunger Position/RConn1
  Solenoid/LConn2 -- Plunger Position/LConn1
  2+/RConn1 -- Microswitch/LConn1
  Microswitch/RConn2 -- 2-/RConn1
  Plunger Position/RConn3 -- Clutch/LConn2 -- Plunger to lever extension conversion/LConn1
  Plunger to lever extension conversion/RConn1 -- Microswitch/RConn1
  Clutch/LConn1 -- C/RConn1
  R/RConn1 -- Clutch/RConn1

== system TraditionalStarterGenerator/Subsystem ==
  Simulink-PS Converter : nesl_utility/Simulink-PS Converter  PhysicalDomain=network_engine_domain  SubClassName=ps_input  LeftPortType=input  RightPortType=output  PseudoPeriodic=off  Frequencies=[]  NoiseDistribution=none  NoiseParameters=[]  Unit=1  AffineConversion=off  FilteringAndDerivatives=zero  SimscapeFilterOrder=1  InputFilterTimeConstant=0.001  UdotUserProvided=1
  ignition : PMIOPort  Side=Right
  wires:
  [ignition] -> Simulink-PS Converter/1
  connections:
  Simulink-PS Converter/RConn1 -- ignition/RConn1

== system TraditionalStarterGenerator/Subsystem1 ==
  Simulink-PS Converter : nesl_utility/Simulink-PS Converter  PhysicalDomain=network_engine_domain  SubClassName=ps_input  LeftPortType=input  RightPortType=output  PseudoPeriodic=off  Frequencies=[]  NoiseDistribution=none  NoiseParameters=[]  Unit=1  AffineConversion=off  FilteringAndDerivatives=zero  SimscapeFilterOrder=1  InputFilterTimeConstant=0.001  UdotUserProvided=1
  starter : PMIOPort  Side=Right
  wires:
  [starter] -> Simulink-PS Converter/1
  connections:
  Simulink-PS Converter/RConn1 -- starter/RConn1

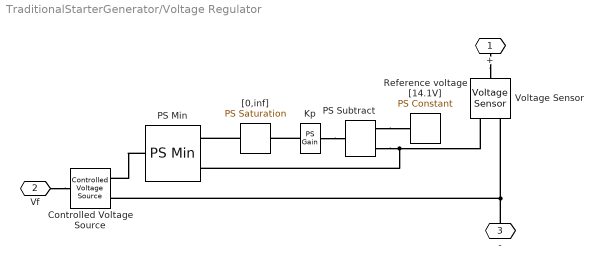
== system TraditionalStarterGenerator/Voltage Regulator ==
  Controlled Voltage Source : fl_lib/Electrical/Electrical Sources/Controlled Voltage Source
  Kp : fl_ps_legacy_lib/Legacy Physical Signals/Functions/PS Gain  gain=100
  PS Min : fl_ps_legacy_lib/Legacy Physical Signals/Nonlinear Operators/PS Min
      settings: InternalSimscapePortConfiguration="{\"Bottom\":[],\"Left\":[{\"id\":\"I1\",\"label\":\"\",\"type\":\"input\"},{\"id\":\"I2\",\"label\":\"\",\"type\":\"input\"}],\"Right\":[{\"id\":\"O\",\"label\":\"\",\"type\":\"output\"}],\"Top\":[]}"
  PS Subtract : fl_ps_legacy_lib/Legacy Physical Signals/Functions/PS Subtract
  Reference voltage [14.1V] : fl_lib/Physical Signals/Sources/PS Constant  constant=14.1
  Voltage Sensor : fl_lib/Electrical/Electrical Sensors/Voltage Sensor
  "[0,inf]" : fl_ps_legacy_lib/Legacy Physical Signals/Nonlinear Operators/PS Saturation  upper_limit=inf  lower_limit=0
      settings: InternalSimscapePortConfiguration="{\"Bottom\":[],\"Left\":[{\"id\":\"I\",\"label\":\"\",\"type\":\"input\"}],\"Right\":[{\"id\":\"O\",\"label\":\"\",\"type\":\"output\"}],\"Top\":[]}"
  + : PMIOPort  Side=Left
  Vf : PMIOPort  Port=2  Side=Right
  - : PMIOPort  Port=3  Side=Left
  connections:
  Kp/LConn1 -- PS Subtract/RConn1
  Kp/RConn1 -- "[0,inf]"/LConn1
  PS Subtract/LConn1 -- Reference voltage [14.1V]/RConn1
  PS Min/LConn1 -- Voltage Sensor/RConn1 -- PS Subtract/LConn2
  +/RConn1 -- Voltage Sensor/LConn1
  -/RConn1 -- Voltage Sensor/RConn2 -- Controlled Voltage Source/RConn2
  "[0,inf]"/RConn1 -- PS Min/LConn2
  PS Min/RConn1 -- Controlled Voltage Source/RConn1
  Vf/RConn1 -- Controlled Voltage Source/LConn1

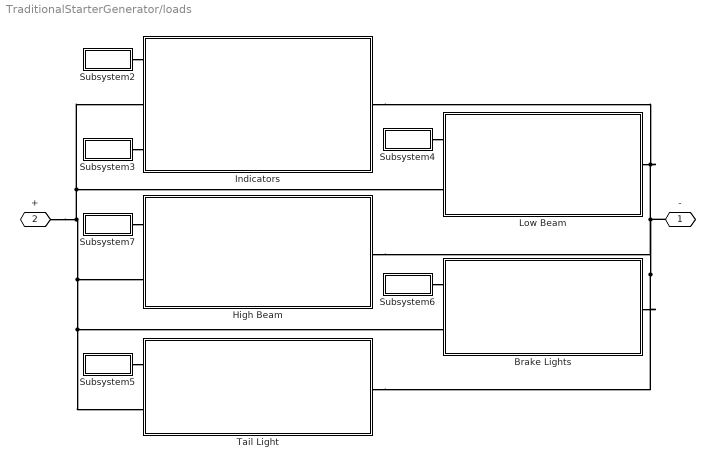
== system TraditionalStarterGenerator/loads ==
  Brake Lights : Subsystem
  High Beam : Subsystem
  Indicators : Subsystem  Tag=PublishSubsystem
  Low Beam : Subsystem
  Subsystem2 : Subsystem
  Subsystem3 : Subsystem
  Subsystem4 : Subsystem
  Subsystem5 : Subsystem
  Subsystem6 : Subsystem
  Subsystem7 : Subsystem
  Tail Light : Subsystem
  - : PMIOPort  Side=Left
  + : PMIOPort  Port=2  Side=Right
  connections:
  Subsystem2/RConn1 -- Indicators/LConn1
  +/RConn1 -- Tail Light/LConn2 -- Brake Lights/LConn2 -- High Beam/LConn2 -- Indicators/LConn2 -- Low Beam/LConn2
  Subsystem3/RConn1 -- Indicators/LConn3
  Subsystem4/RConn1 -- Low Beam/LConn1
  Low Beam/RConn1 -- Indicators/RConn1 -- High Beam/RConn1 -- Tail Light/RConn1 -- Brake Lights/RConn1 -- -/RConn1
  Subsystem7/RConn1 -- High Beam/LConn1
  Subsystem5/RConn1 -- Tail Light/LConn1
  Subsystem6/RConn1 -- Brake Lights/LConn1

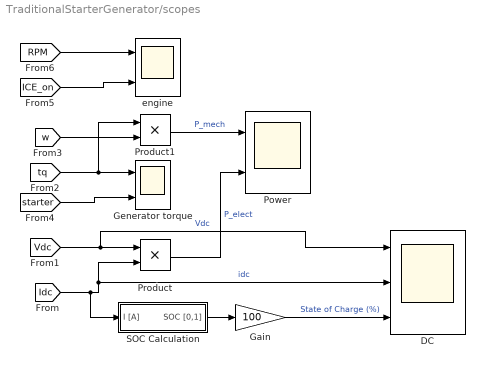
== system TraditionalStarterGenerator/scopes ==
  DC : Scope  NumInputPorts=3
  Gain : Gain  Gain=100
  Generator torque : Scope  NumInputPorts=2
  Power : Scope  NumInputPorts=2
  Product : Product
  Product1 : Product
  SOC Calculation : Subsystem
  engine : Scope  NumInputPorts=2
  wires:
  [RPM] -> engine/1
  [starter] -> Generator torque/2
  [ICE_on] -> engine/2
  [Idc] -> DC/2, Product/2, SOC Calculation/1(I [A])  "idc"
  [w] -> Product1/2
  [tq] -> Product1/1, Generator torque/1
  [Vdc] -> Product/1, DC/1  "Vdc"
  Product1/1 -> Power/1  "P_mech"
  Product/1 -> Power/2  "P_elect"
  SOC Calculation/1(SOC [0,1]) -> Gain/1
  Gain/1 -> DC/3  "State of Charge (%)"

== system TraditionalStarterGenerator/Alternator/Back EMF and Torque ==
  Current Voltage Interface : Subsystem
  Torque Motion Interface : Subsystem
  Torque Voltage Calculations : Subsystem
  R : PMIOPort  Side=Left
  C : PMIOPort  Port=2  Side=Right
  + : PMIOPort  Port=3  Side=Left
  VF : PMIOPort  Port=4  Side=Right
  - : PMIOPort  Port=5  Side=Right
  connections:
  R/RConn1 -- Torque Motion Interface/RConn1
  C/RConn1 -- Torque Motion Interface/LConn1
  Torque Voltage Calculations/LConn1 -- Torque Motion Interface/RConn2
  Torque Motion Interface/LConn2 -- Torque Voltage Calculations/LConn2
  VF/RConn1 -- Torque Voltage Calculations/LConn3
  +/RConn1 -- Current Voltage Interface/LConn2
  Current Voltage Interface/LConn1 -- Torque Voltage Calculations/RConn1
  Current Voltage Interface/RConn1 -- Torque Voltage Calculations/RConn2
  -/RConn1 -- Current Voltage Interface/RConn2

== system TraditionalStarterGenerator/Starter Solenoid/Clutch ==
  -1 : fl_ps_legacy_lib/Legacy Physical Signals/Functions/PS Gain  gain=-1
  Engage : Subsystem
  Motion Sensor : fl_lib/Mechanical/Mechanical Sensors/Ideal Rotational Motion Sensor  reference=foundation.enum.MeasurementReference.difference  acceleration_port=false  velocity_port=true  position_port=true  wrap_angle=simscape.enum.onoff.off  offset=0 rad
  Torque Source : fl_lib/Mechanical/Mechanical Sources/Ideal Torque Source
  kw : fl_ps_legacy_lib/Legacy Physical Signals/Functions/PS Product
  R : PMIOPort  Side=Left
  S : PMIOPort  Port=2  Side=Left
  C : PMIOPort  Port=3  Side=Right
  connections:
  Torque Source/LConn1 -- Motion Sensor/LConn1 -- R/RConn1
  C/RConn1 -- Motion Sensor/RConn1 -- Torque Source/RConn2
  Motion Sensor/RConn2 -- -1/LConn1
  kw/RConn1 -- Torque Source/RConn1
  -1/RConn1 -- kw/LConn2
  S/RConn1 -- Engage/LConn1
  Engage/RConn1 -- kw/LConn1

== system TraditionalStarterGenerator/loads/Brake Lights ==
  Fuse : ee_lib/Switches & Breakers/Fuse  prm=1  I_rated=10 A  melt_margin=1  T_fuse=0.5 s  I2t=1 s*A^2  I_vec=[1.9, 2.0, 2.5, 30.0] A  t_vec=[10000.0, 1.0, 0.3, 0.001] s  R_closed=0.01 Ohm  G_open=1e-8 1/Ohm  exposemeasurement=ee.enum.exposemeasurement.hidden
      settings: AttributesFormatString=%<I_rated> %<I_rated_unit>  InternalSimscapePortConfiguration="{\"Bottom\":[],\"Left\":[{\"id\":\"p\",\"label\":\"\",\"type\":\"foundation.electrical.electrical\"}],\"Right\":[{\"id\":\"n\",\"label\":\"\",\"type\":\"foundation.electrical.electrical\"}],\"Top\":[]}"
  Lamp Right : ee_lib/Passive/Incandescent Lamp  R_param=2  R0=0.15 Ohm  R1=1 Ohm  i0=5*3/12 A  i1=3/12 A  Vrated=12 V  alpha=0.004 1/K  tc=25 ms  initial_state=simscape.enum.onoff.off  t_fault=inf s
      settings: InternalSimscapePortConfiguration="{\"Bottom\":[],\"Left\":[{\"id\":\"p\",\"label\":\"+\",\"type\":\"foundation.electrical.electrical\"}],\"Right\":[{\"id\":\"n\",\"label\":\"-\",\"type\":\"foundation.electrical.electrical\"}],\"Top\":[]}"
  Switch SPST : ee_lib/Switches & Breakers/SPST Switch  R_closed=1 Ohm  G_open=1e-6 S  Threshold=0.5 V  Width=0 V  model_dynamics=0  t_on=0.001 s  t_off=0.001 s  initial_vT=0 V
      settings: InternalSimscapePortConfiguration="{\"Bottom\":[],\"Left\":[{\"id\":\"vT\",\"label\":\"vT\",\"type\":\"input\"},{\"id\":\"p\",\"label\":\"\",\"type\":\"foundation.electrical.electrical\"}],\"Right\":[{\"id\":\"n\",\"label\":\"\",\"type\":\"foundation.electrical.electrical\"}],\"Top\":[]}"
  Switch : PMIOPort  Side=Left
  + : PMIOPort  Port=2  Side=Left
  - : PMIOPort  Port=3  Side=Right
  connections:
  Lamp Right/RConn1 -- -/RConn1
  +/RConn1 -- Fuse/LConn1
  Fuse/RConn1 -- Switch SPST/LConn2
  Switch SPST/RConn1 -- Lamp Right/LConn1
  Switch/RConn1 -- Switch SPST/LConn1

== system TraditionalStarterGenerator/loads/High Beam ==
  Fuse Left : ee_lib/Switches & Breakers/Fuse  prm=1  I_rated=10 A  melt_margin=1  T_fuse=0.5 s  I2t=1 s*A^2  I_vec=[1.9, 2.0, 2.5, 30.0] A  t_vec=[10000.0, 1.0, 0.3, 0.001] s  R_closed=0.01 Ohm  G_open=1e-8 1/Ohm  exposemeasurement=ee.enum.exposemeasurement.hidden
      settings: AttributesFormatString=%<I_rated> %<I_rated_unit>  InternalSimscapePortConfiguration="{\"Bottom\":[],\"Left\":[{\"id\":\"p\",\"label\":\"\",\"type\":\"foundation.electrical.electrical\"}],\"Right\":[{\"id\":\"n\",\"label\":\"\",\"type\":\"foundation.electrical.electrical\"}],\"Top\":[]}"
  Lamp : ee_lib/Passive/Incandescent Lamp  R_param=2  R0=0.15 Ohm  R1=1 Ohm  i0=5*20/12 A  i1=20/12 A  Vrated=12 V  alpha=0.004 1/K  tc=25 ms  initial_state=simscape.enum.onoff.off  t_fault=inf s
      settings: InternalSimscapePortConfiguration="{\"Bottom\":[],\"Left\":[{\"id\":\"p\",\"label\":\"+\",\"type\":\"foundation.electrical.electrical\"}],\"Right\":[{\"id\":\"n\",\"label\":\"-\",\"type\":\"foundation.electrical.electrical\"}],\"Top\":[]}"
  SPST Switch : ee_lib/Switches & Breakers/SPST Switch  R_closed=0.01 Ohm  G_open=1e-6 S  Threshold=0.5 V  Width=0 V  model_dynamics=0  t_on=1e-3 s  t_off=1e-3 s  initial_vT=0 V
      settings: InternalSimscapePortConfiguration="{\"Bottom\":[],\"Left\":[{\"id\":\"vT\",\"label\":\"vT\",\"type\":\"input\"},{\"id\":\"p\",\"label\":\"\",\"type\":\"foundation.electrical.electrical\"}],\"Right\":[{\"id\":\"n\",\"label\":\"\",\"type\":\"foundation.electrical.electrical\"}],\"Top\":[]}"
  Switch : PMIOPort  Side=Left
  + : PMIOPort  Port=2  Side=Left
  - : PMIOPort  Port=3  Side=Right
  connections:
  Lamp/RConn1 -- -/RConn1
  Fuse Left/LConn1 -- +/RConn1
  SPST Switch/LConn2 -- Fuse Left/RConn1
  Lamp/LConn1 -- SPST Switch/RConn1
  Switch/RConn1 -- SPST Switch/LConn1

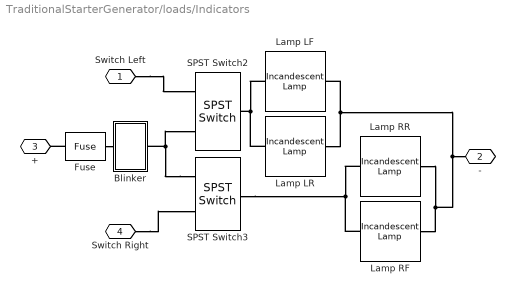
== system TraditionalStarterGenerator/loads/Indicators ==
  Blinker : Subsystem
  Fuse : ee_lib/Switches & Breakers/Fuse  prm=1  I_rated=10 A  melt_margin=1  T_fuse=0.5 s  I2t=1 s*A^2  I_vec=[1.9, 2.0, 2.5, 30.0] A  t_vec=[10000.0, 1.0, 0.3, 0.001] s  R_closed=0.01 Ohm  G_open=1e-8 1/Ohm  exposemeasurement=ee.enum.exposemeasurement.hidden
      settings: AttributesFormatString=%<I_rated> %<I_rated_unit>  InternalSimscapePortConfiguration="{\"Bottom\":[],\"Left\":[{\"id\":\"p\",\"label\":\"\",\"type\":\"foundation.electrical.electrical\"}],\"Right\":[{\"id\":\"n\",\"label\":\"\",\"type\":\"foundation.electrical.electrical\"}],\"Top\":[]}"
  Lamp LF : ee_lib/Passive/Incandescent Lamp  R_param=2  R0=0.15 Ohm  R1=1 Ohm  i0=5*3/12 A  i1=3/12 A  Vrated=12 V  alpha=0.004 1/K  tc=25 ms  initial_state=simscape.enum.onoff.off  t_fault=inf s
      settings: InternalSimscapePortConfiguration="{\"Bottom\":[],\"Left\":[{\"id\":\"p\",\"label\":\"+\",\"type\":\"foundation.electrical.electrical\"}],\"Right\":[{\"id\":\"n\",\"label\":\"-\",\"type\":\"foundation.electrical.electrical\"}],\"Top\":[]}"
  Lamp LR : ee_lib/Passive/Incandescent Lamp  R_param=2  R0=0.15 Ohm  R1=1 Ohm  i0=5*3/12 A  i1=3/12 A  Vrated=12 V  alpha=0.004 1/K  tc=25 ms  initial_state=simscape.enum.onoff.off  t_fault=inf s
      settings: InternalSimscapePortConfiguration="{\"Bottom\":[],\"Left\":[{\"id\":\"p\",\"label\":\"+\",\"type\":\"foundation.electrical.electrical\"}],\"Right\":[{\"id\":\"n\",\"label\":\"-\",\"type\":\"foundation.electrical.electrical\"}],\"Top\":[]}"
  Lamp RF : ee_lib/Passive/Incandescent Lamp  R_param=2  R0=0.15 Ohm  R1=1 Ohm  i0=5*3/12 A  i1=3/12 A  Vrated=12 V  alpha=0.004 1/K  tc=25 ms  initial_state=simscape.enum.onoff.off  t_fault=inf s
      settings: InternalSimscapePortConfiguration="{\"Bottom\":[],\"Left\":[{\"id\":\"p\",\"label\":\"+\",\"type\":\"foundation.electrical.electrical\"}],\"Right\":[{\"id\":\"n\",\"label\":\"-\",\"type\":\"foundation.electrical.electrical\"}],\"Top\":[]}"
  Lamp RR : ee_lib/Passive/Incandescent Lamp  R_param=2  R0=0.15 Ohm  R1=1 Ohm  i0=5*3/12 A  i1=3/12 A  Vrated=12 V  alpha=0.004 1/K  tc=25 ms  initial_state=simscape.enum.onoff.off  t_fault=inf s
      settings: InternalSimscapePortConfiguration="{\"Bottom\":[],\"Left\":[{\"id\":\"p\",\"label\":\"+\",\"type\":\"foundation.electrical.electrical\"}],\"Right\":[{\"id\":\"n\",\"label\":\"-\",\"type\":\"foundation.electrical.electrical\"}],\"Top\":[]}"
  SPST Switch2 : ee_lib/Switches & Breakers/SPST Switch  R_closed=1 Ohm  G_open=1e-6 S  Threshold=0.5 V  Width=0 V  model_dynamics=0  t_on=0.001 s  t_off=0.001 s  initial_vT=0 V
      settings: InternalSimscapePortConfiguration="{\"Bottom\":[],\"Left\":[{\"id\":\"vT\",\"label\":\"vT\",\"type\":\"input\"},{\"id\":\"p\",\"label\":\"\",\"type\":\"foundation.electrical.electrical\"}],\"Right\":[{\"id\":\"n\",\"label\":\"\",\"type\":\"foundation.electrical.electrical\"}],\"Top\":[]}"
  SPST Switch3 : ee_lib/Switches & Breakers/SPST Switch  R_closed=1 Ohm  G_open=1e-6 S  Threshold=0.5 V  Width=0 V  model_dynamics=0  t_on=0.001 s  t_off=0.001 s  initial_vT=0 V
      settings: InternalSimscapePortConfiguration="{\"Bottom\":[],\"Left\":[{\"id\":\"vT\",\"label\":\"vT\",\"type\":\"input\"},{\"id\":\"p\",\"label\":\"\",\"type\":\"foundation.electrical.electrical\"}],\"Right\":[{\"id\":\"n\",\"label\":\"\",\"type\":\"foundation.electrical.electrical\"}],\"Top\":[]}"
  Switch Left : PMIOPort  Side=Left
  - : PMIOPort  Port=2  Side=Right
  + : PMIOPort  Port=3  Side=Left
  Switch Right : PMIOPort  Port=4  Side=Left
  connections:
  Lamp RR/RConn1 -- Lamp LR/RConn1 -- Lamp LF/RConn1 -- -/RConn1 -- Lamp RF/RConn1
  Switch Right/RConn1 -- SPST Switch3/LConn1
  Switch Left/RConn1 -- SPST Switch2/LConn1
  Lamp LR/LConn1 -- Lamp LF/LConn1 -- SPST Switch2/RConn1
  Lamp RR/LConn1 -- Lamp RF/LConn1 -- SPST Switch3/RConn1
  SPST Switch3/LConn2 -- SPST Switch2/LConn2 -- Blinker/RConn1
  Fuse/RConn1 -- Blinker/LConn1
  Fuse/LConn1 -- +/RConn1
